simulink model "NeuromuscularModelwReflex2"  (R2019b)
settings: Solver=ode15s  StartTime=0.0  StopTime=20  MaxStep=.01  RelTol=1e-4  AbsTol=1e-6  EnableMultiTasking=on
undefined symbols (not defined in the file): footCenterToCGDist, footInertia, footMass, g, LceOffsetTA, legAngleTgt, LlegLengthClr, LongDelay, loptGAS, loptHAM, loptHAMCut, loptTA, lslackGAS, lslackHAM, lslackHAMCut, MidDelay, phimaxGASa, phimaxGASk, phimaxHAMk, phirefGASa, phirefGASk, phirefHAMh, phirefHAMk, rGASa, rGASk, rHAMh, rHAMk, rhoGASa, rhoGASk, rhoHAMh, rhoHAMk, RlegLengthClr, ShortDelay, simbiconGainD, simbiconGainV, simbiconLegAngle0, X, Y, Z
libraries: NeuroMuscularLibrary x81, nesl_utility x16, sm_lib x14, simulink x5, simulink_extras x2
(part 2 of 2)

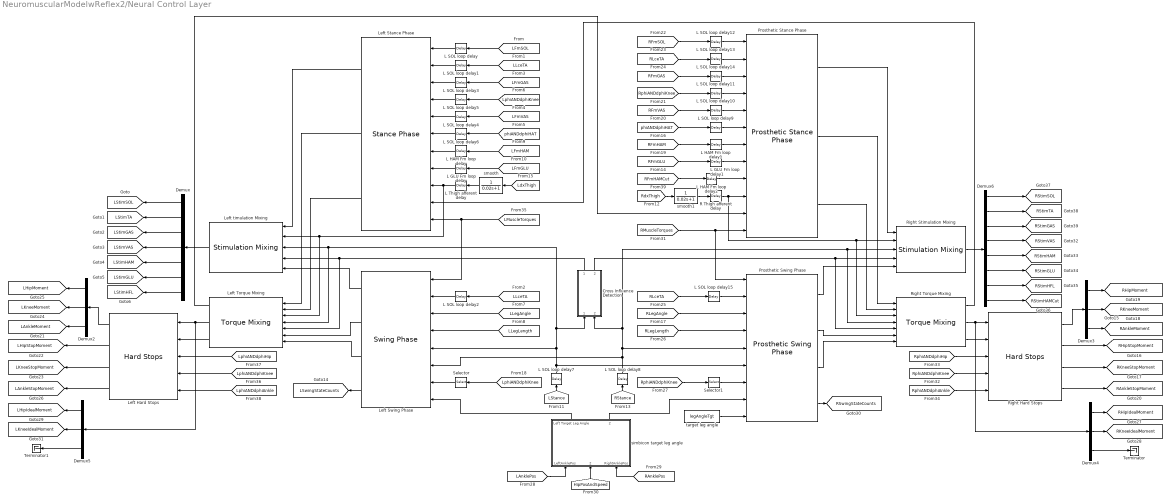
== system NeuromuscularModelwReflex2/Neural Control Layer ==
  Cross Influence Detection : Subsystem
  Demux : Demux  Outputs=7
  Demux{2..5} (4 alike) : Demux  Outputs=3
  Demux6 : Demux  Outputs=8
  L GLU Fm loop delay : TransportDelay  DelayTime=ShortDelay
  L GLU Fm loop delay1 : TransportDelay  DelayTime=ShortDelay
  L HAM Fm loop delay : TransportDelay  DelayTime=ShortDelay
  L HAM Fm loop delay1 : TransportDelay  DelayTime=ShortDelay
  L HAM Fm loop delay2 : TransportDelay  DelayTime=ShortDelay  BufferSize=2048
  L SOL loop delay{,1..3,12..15} (8 alike) : TransportDelay  DelayTime=LongDelay
  L SOL loop delay{4..5,7..8,10..11} (6 alike) : TransportDelay  DelayTime=MidDelay
  L SOL loop delay6 : TransportDelay  DelayTime=ShortDelay
  L SOL loop delay9 : TransportDelay  DelayTime=ShortDelay
  L Thigh afferent delay : TransportDelay  DelayTime=ShortDelay
  Left Hard Stops : NeuroMuscularLibrary/Hard Stops  SystemSampleTime=-1  Latency=0  AutoFrameSizeCalculation=off
  Left Stance Phase : NeuroMuscularLibrary/Stance Phase  GainHAM=LGainHAM  GainGLU=LGainGLU  GainSOL=LGainSOL  GainSOLTA=LGainSOLTA  GainTA=LGainTA  GainGAS=LGainGAS  GainVAS=LGainVAS  GainKneeOverExt=LGainKneeOverExt  PosGainGG=LPosGainGG  SpeedGainGG=LSpeedGainGG  Kglu=LKglu
  Left Swing Phase : NeuroMuscularLibrary/Swing Phase  GainTA=LGainTA  hipPGain=LhipPGain  hipDGain=LhipDGain  legAngleFilter=LlegAngleFilter  kneeFlexGain=LkneeFlexGain  kneeHoldGain1=LkneeHoldGain1  kneeHoldGain2=LkneeHoldGain2  kneeStopGain=LkneeStopGain  kneeExtendGain=LkneeExtendGain  legLengthClr=LlegLengthClr
  Left Torque Mixing : NeuroMuscularLibrary/Torque Mixing  SystemSampleTime=-1  Latency=0  AutoFrameSizeCalculation=off
  Left timulation Mixing : NeuroMuscularLibrary/Stimulation Mixing  SystemSampleTime=-1  Latency=0  AutoFrameSizeCalculation=off
  Prosthetic Stance Phase : NeuroMuscularLibrary/Prosthetic Stance Phase  GainHAM=RGainHAM  GainHAMCut=RGainHAMCut  GainGLU=RGainGLU  GainSOL=RGainSOL  GainSOLTA=RGainSOLTA  GainTA=RGainTA  GainGAS=RGainGAS  GainVAS=RGainVAS  GainKneeOverExt=RGainKneeOverExt  PosGainGG=RPosGainGG  SpeedGainGG=RSpeedGainGG  Kglu=RKglu
  Prosthetic Swing Phase : NeuroMuscularLibrary/Prosthetic Swing Phase  GainTA=RGainTA  hipPGain=RhipPGain  hipDGain=RhipDGain  legAngleFilter=RlegAngleFilter  kneeFlexGain=RkneeFlexGain  kneeHoldGain1=RkneeHoldGain1  kneeHoldGain2=RkneeHoldGain2  kneeStopGain=RkneeStopGain  kneeExtendGain=RkneeExtendGain  legLengthClr=RlegLengthClr
  R Thigh afferent delay : TransportDelay  DelayTime=ShortDelay
  Right Hard Stops : NeuroMuscularLibrary/Hard Stops  SystemSampleTime=-1  Latency=0  AutoFrameSizeCalculation=off
  Right Stimulation Mixing : NeuroMuscularLibrary/Stimulation Mixing  SystemSampleTime=-1  Latency=0  AutoFrameSizeCalculation=off
  Right Torque Mixing : NeuroMuscularLibrary/Torque Mixing  SystemSampleTime=-1  Latency=0  AutoFrameSizeCalculation=off
  Selector : Selector  InputPortWidth=2  IndexOptions=Index vector (dialog)  Indices=2  OutputSizes=1
  Selector1 : Selector  InputPortWidth=2  IndexOptions=Index vector (dialog)  Indices=2  OutputSizes=1
  Terminator : Terminator
  Terminator1 : Terminator
  simbicon target leg angle : Subsystem
  smooth : TransferFcn  Denominator=[0.02 1]
  smooth1 : TransferFcn  Denominator=[0.02 1]
  target leg angle : Constant  Value=legAngleTgt
  tag scope: LAnkleMoment=global, LAnkleStopMoment=global, LHipIdealMoment=global, LHipMoment=global, LHipStopMoment=global, LKneeIdealMoment=global, LKneeMoment=global, LKneeStopMoment=global, LStimGAS=global, LStimGLU=global, LStimHAM=global, LStimHFL=global, LStimSOL=global, LStimTA=global, LStimVAS=global, LSwingStateCounts=global, RAnkleMoment=global, RAnkleStopMoment=global, RHipIdealMoment=global, RHipMoment=global, RHipStopMoment=global, RKneeIdealMoment=global, RKneeMoment=global, RKneeStopMoment=global, RStimGAS=global, RStimGLU=global, RStimHAM=global, RStimHAMCut=global, RStimHFL=global, RStimSOL=global, RStimTA=global, RStimVAS=global, RSwingStateCounts=global
  wires:
  [LFmSOL] -> L SOL loop delay/1
  L SOL loop delay/1 -> Left Stance Phase/1
  [LLceTA] -> L SOL loop delay1/1
  L SOL loop delay1/1 -> Left Stance Phase/2
  Demux/1 -> [LStimSOL]
  Demux/2 -> [LStimTA]
  Demux/3 -> [LStimGAS]
  [LFmGAS] -> L SOL loop delay3/1
  L SOL loop delay3/1 -> Left Stance Phase/3
  [LLceTA] -> L SOL loop delay2/1
  L SOL loop delay4/1 -> Left Stance Phase/5
  [LFmVAS] -> L SOL loop delay4/1
  L SOL loop delay5/1 -> Left Stance Phase/4
  [LphiANDdphiKnee] -> L SOL loop delay5/1
  Demux/4 -> [LStimVAS]
  [phiANDdphiHAT] -> L SOL loop delay6/1
  L SOL loop delay6/1 -> Left Stance Phase/6
  Demux/5 -> [LStimHAM]
  Demux/6 -> [LStimGLU]
  Demux/7 -> [LStimHFL]
  [LdxThigh] -> smooth/1
  smooth/1 -> L Thigh afferent delay/1
  [RdxThigh] -> smooth1/1
  smooth1/1 -> R Thigh afferent delay/1
  [LFmHAM] -> L HAM Fm loop delay/1
  [LFmGLU] -> L GLU Fm loop delay/1
  L SOL loop delay7/1 -> Prosthetic Swing Phase/6, Left Swing Phase/5, Left Torque Mixing/4, Left timulation Mixing/3, Cross Influence Detection/1(LStance)
  [RFmHAM] -> L HAM Fm loop delay1/1
  [RFmGLU] -> L GLU Fm loop delay1/1
  [phiANDdphiHAT] -> L SOL loop delay9/1
  L SOL loop delay9/1 -> Prosthetic Stance Phase/6
  [LStance] -> L SOL loop delay7/1
  [RStance] -> L SOL loop delay8/1
  [RFmVAS] -> L SOL loop delay10/1
  [RphiANDdphiKnee] -> L SOL loop delay11/1
  L SOL loop delay10/1 -> Prosthetic Stance Phase/5
  L SOL loop delay11/1 -> Prosthetic Stance Phase/4
  L SOL loop delay12/1 -> Prosthetic Stance Phase/1
  [RFmSOL] -> L SOL loop delay12/1
  [RLceTA] -> L SOL loop delay13/1
  L SOL loop delay13/1 -> Prosthetic Stance Phase/2
  [RFmGAS] -> L SOL loop delay14/1
  L SOL loop delay14/1 -> Prosthetic Stance Phase/3
  [RLceTA] -> L SOL loop delay15/1
  L Thigh afferent delay/1 -> Left Torque Mixing/3, Left timulation Mixing/2, Left Stance Phase/9
  L HAM Fm loop delay/1 -> Left Stance Phase/7
  L GLU Fm loop delay/1 -> Left Stance Phase/8
  R Thigh afferent delay/1 -> Prosthetic Stance Phase/10, Right Torque Mixing/3, Right Stimulation Mixing/2
  L SOL loop delay15/1 -> Prosthetic Swing Phase/2
  L SOL loop delay2/1 -> Left Swing Phase/2
  Prosthetic Stance Phase/1 -> Right Stimulation Mixing/1
  L SOL loop delay8/1 -> Left Swing Phase/6, Prosthetic Swing Phase/5, Right Torque Mixing/4, Right Stimulation Mixing/3, Cross Influence Detection/2(RStance)
  Cross Influence Detection/2(LeftLeading) -> Right Torque Mixing/5, Right Stimulation Mixing/4
  Left timulation Mixing/1 -> Demux/1
  Left Stance Phase/1 -> Left timulation Mixing/1
  Cross Influence Detection/1(RightLeading) -> Left Torque Mixing/5, Left timulation Mixing/4
  Demux3/1 -> [RHipMoment]
  Demux3/2 -> [RKneeMoment]
  [LLegAngle] -> Left Swing Phase/3
  [LLegLength] -> Left Swing Phase/4
  [RLegAngle] -> Prosthetic Swing Phase/3
  [RLegLength] -> Prosthetic Swing Phase/4
  [RphiANDdphiKnee] -> Selector1/1
  Selector1/1 -> Prosthetic Swing Phase/7
  [LAnklePos] -> simbicon target leg angle/1(LeftAnklePos)
  [RAnklePos] -> simbicon target leg angle/3(RightAnklePos)
  Prosthetic Swing Phase/1 -> Right Stimulation Mixing/5
  [LphiANDdphiKnee] -> Selector/1
  Selector/1 -> Left Swing Phase/7
  Left Swing Phase/1 -> Left timulation Mixing/5
  [HipPosAndSpeed] -> simbicon target leg angle/2(HIPposAndSpeed)
  simbicon target leg angle/2(Right Target Leg Angle) -> Prosthetic Swing Phase/8
  simbicon target leg angle/1(Left Target Leg Angle) -> Left Swing Phase/8
  Prosthetic Swing Phase/4 -> [RSwingStateCounts]
  Left Swing Phase/4 -> [LSwingStateCounts]
  Demux3/3 -> [RAnkleMoment]
  [RphiANDdphiKnee] -> Right Hard Stops/4
  [RphiANDdphiHip] -> Right Hard Stops/3
  [RphiANDdphiAnkle] -> Right Hard Stops/5
  Right Hard Stops/2 -> [RHipStopMoment]
  Right Hard Stops/3 -> [RKneeStopMoment]
  Right Hard Stops/4 -> [RAnkleStopMoment]
  [LMuscleTorques] -> Left Swing Phase/1, Left Stance Phase/11
  Demux2/1 -> [LHipMoment]
  Demux2/3 -> [LAnkleMoment]
  Left Hard Stops/1 -> Demux2/1
  [LphiANDdphiKnee] -> Left Hard Stops/4
  [LphiANDdphiHip] -> Left Hard Stops/3
  Left Hard Stops/2 -> [LHipStopMoment]
  Left Hard Stops/3 -> [LKneeStopMoment]
  Left Hard Stops/4 -> [LAnkleStopMoment]
  Left Stance Phase/2 -> Left Torque Mixing/1
  Demux2/2 -> [LKneeMoment]
  Right Torque Mixing/2 -> Demux4/1, Right Hard Stops/1
  Right Hard Stops/1 -> Demux3/1
  [RMuscleTorques] -> Prosthetic Stance Phase/12, Prosthetic Swing Phase/1
  Demux4/1 -> [RHipIdealMoment]
  Demux4/2 -> [RKneeIdealMoment]
  Demux4/3 -> Terminator/1
  Prosthetic Swing Phase/3 -> Right Torque Mixing/7
  Prosthetic Swing Phase/2 -> Right Torque Mixing/6
  Prosthetic Stance Phase/3 -> Right Torque Mixing/2
  Prosthetic Stance Phase/2 -> Right Torque Mixing/1
  Right Torque Mixing/3 -> Right Hard Stops/2
  Right Torque Mixing/1 -> Left Stance Phase/10
  [LphiANDdphiAnkle] -> Left Hard Stops/5
  Left Torque Mixing/2 -> Demux5/1, Left Hard Stops/1
  Left Torque Mixing/3 -> Left Hard Stops/2
  Left Torque Mixing/1 -> Prosthetic Stance Phase/11
  Left Stance Phase/3 -> Left Torque Mixing/2
  Left Swing Phase/2 -> Left Torque Mixing/6
  Left Swing Phase/3 -> Left Torque Mixing/7
  Demux5/1 -> [LHipIdealMoment]
  Demux5/2 -> [LKneeIdealMoment]
  Demux5/3 -> Terminator1/1
  Demux6/1 -> [RStimSOL]
  Demux6/2 -> [RStimTA]
  Demux6/4 -> [RStimVAS]
  Demux6/5 -> [RStimHAM]
  Demux6/7 -> [RStimHFL]
  Demux6/3 -> [RStimGAS]
  Demux6/6 -> [RStimGLU]
  Right Stimulation Mixing/1 -> Demux6/1
  Demux6/8 -> [RStimHAMCut]
  L HAM Fm loop delay1/1 -> Prosthetic Stance Phase/7
  L GLU Fm loop delay1/1 -> Prosthetic Stance Phase/8
  [RFmHAMCut] -> L HAM Fm loop delay2/1
  L HAM Fm loop delay2/1 -> Prosthetic Stance Phase/9
  target leg angle/1 -> Prosthetic Swing Phase/9

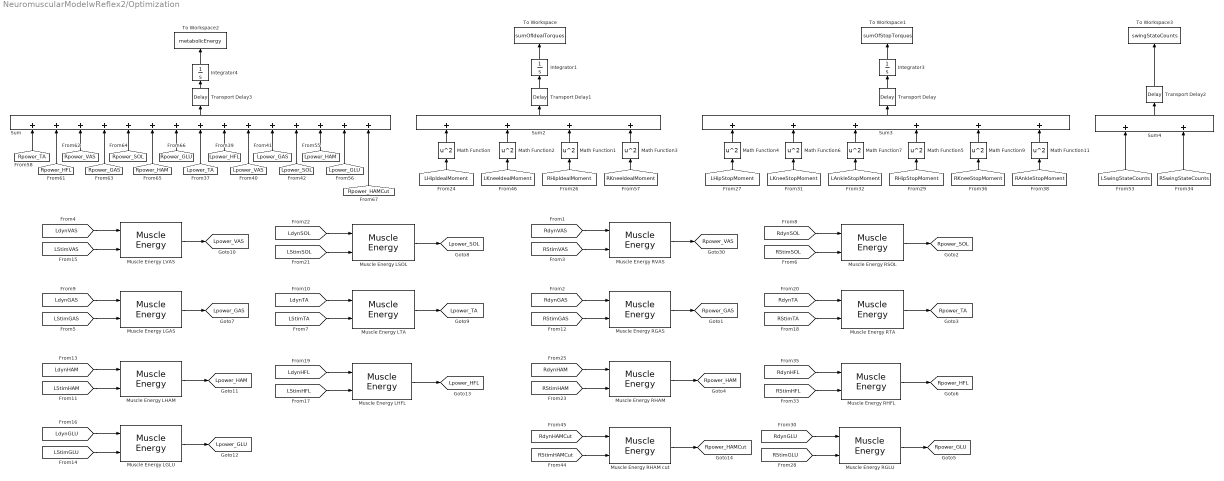
== system NeuromuscularModelwReflex2/Optimization ==
  Integrator1 : Integrator
  Integrator3 : Integrator
  Integrator4 : Integrator
  Math Function{,1..7,9,11} (10 alike) : Math  Operator=square  SaturateOnIntegerOverflow=on
  Muscle Energy LGAS : NeuroMuscularLibrary/Muscle Energy  lopt=loptGAS  FT=FT_GAS  Fmax=FmaxGAS
  Muscle Energy LGLU : NeuroMuscularLibrary/Muscle Energy  lopt=loptGLU  FT=FT_GLU  Fmax=FmaxGLU
  Muscle Energy LHAM : NeuroMuscularLibrary/Muscle Energy  lopt=loptHAM  FT=FT_HAM  Fmax=FmaxHAM
  Muscle Energy LHFL : NeuroMuscularLibrary/Muscle Energy  lopt=loptHFL  FT=FT_HFL  Fmax=FmaxHFL
  Muscle Energy LSOL : NeuroMuscularLibrary/Muscle Energy  lopt=loptSOL  FT=FT_SOL  Fmax=FmaxSOL
  Muscle Energy LTA : NeuroMuscularLibrary/Muscle Energy  lopt=loptTA  FT=FT_TA  Fmax=FmaxTA
  Muscle Energy LVAS : NeuroMuscularLibrary/Muscle Energy  lopt=loptVAS  FT=FT_VAS  Fmax=FmaxVAS
  Muscle Energy RGAS : NeuroMuscularLibrary/Muscle Energy  lopt=loptGAS  FT=FT_GAS  Fmax=FmaxGAS
  Muscle Energy RGLU : NeuroMuscularLibrary/Muscle Energy  lopt=loptGLU  FT=FT_GLU  Fmax=FmaxGLU
  Muscle Energy RHAM : NeuroMuscularLibrary/Muscle Energy  lopt=loptHAM  FT=FT_HAM  Fmax=FmaxHAM
  Muscle Energy RHAM cut : NeuroMuscularLibrary/Muscle Energy  lopt=loptHAMCut  FT=FT_HAM  Fmax=FmaxHAMCut
  Muscle Energy RHFL : NeuroMuscularLibrary/Muscle Energy  lopt=loptHFL  FT=FT_HFL  Fmax=FmaxHFL
  Muscle Energy RSOL : NeuroMuscularLibrary/Muscle Energy  lopt=loptSOL  FT=FT_SOL  Fmax=FmaxSOL
  Muscle Energy RTA : NeuroMuscularLibrary/Muscle Energy  lopt=loptTA  FT=FT_TA  Fmax=FmaxTA
  Muscle Energy RVAS : NeuroMuscularLibrary/Muscle Energy  lopt=loptVAS  FT=FT_VAS  Fmax=FmaxVAS
  Sum : Sum  Inputs=+++++++++++++++
  Sum2 : Sum  Inputs=++++
  Sum3 : Sum  Inputs=++++++
  Sum4 : Sum
  To Workspace : ToWorkspace  VariableName=sumOfIdealTorques  SampleTime=-1
      settings: MaxDataPoints=1
  To Workspace1 : ToWorkspace  VariableName=sumOfStopTorques  SampleTime=-1
      settings: MaxDataPoints=1
  To Workspace2 : ToWorkspace  VariableName=metabolicEnergy  SampleTime=-1
      settings: MaxDataPoints=1
  To Workspace3 : ToWorkspace  VariableName=swingStateCounts  SampleTime=-1
      settings: MaxDataPoints=1
  Transport Delay{,1..3} (4 alike) : TransportDelay  DelayTime=3  BufferSize=24576
  tag scope: Lpower_GAS=global, Lpower_GLU=global, Lpower_HAM=global, Lpower_HFL=global, Lpower_SOL=global, Lpower_TA=global, Lpower_VAS=global, Rpower_GAS=global, Rpower_GLU=global, Rpower_HAM=global, Rpower_HAMCut=global, Rpower_HFL=global, Rpower_SOL=global, Rpower_TA=global, Rpower_VAS=global
  wires:
  [RdynSOL] -> Muscle Energy RSOL/1
  [RStimSOL] -> Muscle Energy RSOL/2
  [RStimVAS] -> Muscle Energy RVAS/2
  [RStimGAS] -> Muscle Energy RGAS/2
  Muscle Energy RVAS/1 -> [Rpower_VAS]
  Muscle Energy RGAS/1 -> [Rpower_GAS]
  Muscle Energy RSOL/1 -> [Rpower_SOL]
  Muscle Energy RTA/1 -> [Rpower_TA]
  [RdynTA] -> Muscle Energy RTA/1
  [RStimTA] -> Muscle Energy RTA/2
  [RdynHAM] -> Muscle Energy RHAM/1
  [RStimHAM] -> Muscle Energy RHAM/2
  [RdynGLU] -> Muscle Energy RGLU/1
  [RStimGLU] -> Muscle Energy RGLU/2
  [RdynHFL] -> Muscle Energy RHFL/1
  [RStimHFL] -> Muscle Energy RHFL/2
  Muscle Energy RHAM/1 -> [Rpower_HAM]
  Muscle Energy RGLU/1 -> [Rpower_GLU]
  Muscle Energy RHFL/1 -> [Rpower_HFL]
  [RdynGAS] -> Muscle Energy RGAS/1
  [RdynVAS] -> Muscle Energy RVAS/1
  [LdynSOL] -> Muscle Energy LSOL/1
  [LStimSOL] -> Muscle Energy LSOL/2
  [LStimVAS] -> Muscle Energy LVAS/2
  [LStimGAS] -> Muscle Energy LGAS/2
  Muscle Energy LVAS/1 -> [Lpower_VAS]
  Muscle Energy LGAS/1 -> [Lpower_GAS]
  Muscle Energy LSOL/1 -> [Lpower_SOL]
  Muscle Energy LTA/1 -> [Lpower_TA]
  [LdynTA] -> Muscle Energy LTA/1
  [LStimTA] -> Muscle Energy LTA/2
  [LdynHAM] -> Muscle Energy LHAM/1
  [LStimHAM] -> Muscle Energy LHAM/2
  [LdynGLU] -> Muscle Energy LGLU/1
  [LStimGLU] -> Muscle Energy LGLU/2
  [LdynHFL] -> Muscle Energy LHFL/1
  [LStimHFL] -> Muscle Energy LHFL/2
  Muscle Energy LHAM/1 -> [Lpower_HAM]
  Muscle Energy LGLU/1 -> [Lpower_GLU]
  Muscle Energy LHFL/1 -> [Lpower_HFL]
  [LdynGAS] -> Muscle Energy LGAS/1
  [LdynVAS] -> Muscle Energy LVAS/1
  [RdynHAMCut] -> Muscle Energy RHAM cut/1
  [RStimHAMCut] -> Muscle Energy RHAM cut/2
  Muscle Energy RHAM cut/1 -> [Rpower_HAMCut]
  Integrator1/1 -> To Workspace/1
  Math Function/1 -> Sum2/1
  [LHipIdealMoment] -> Math Function/1
  Math Function2/1 -> Sum2/2
  [LKneeIdealMoment] -> Math Function2/1
  [RHipIdealMoment] -> Math Function1/1
  Math Function1/1 -> Sum2/3
  [RKneeIdealMoment] -> Math Function3/1
  Math Function3/1 -> Sum2/4
  Integrator3/1 -> To Workspace1/1
  Math Function4/1 -> Sum3/1
  [LHipStopMoment] -> Math Function4/1
  Math Function6/1 -> Sum3/2
  [LKneeStopMoment] -> Math Function6/1
  [RHipStopMoment] -> Math Function5/1
  Math Function7/1 -> Sum3/3
  [LAnkleStopMoment] -> Math Function7/1
  Sum3/1 -> Transport Delay/1
  Transport Delay/1 -> Integrator3/1
  [RKneeStopMoment] -> Math Function9/1
  Math Function9/1 -> Sum3/5
  [RAnkleStopMoment] -> Math Function11/1
  Math Function11/1 -> Sum3/6
  Sum4/1 -> Transport Delay2/1
  Transport Delay2/1 -> To Workspace3/1
  [LSwingStateCounts] -> Sum4/1
  [RSwingStateCounts] -> Sum4/2
  [Rpower_TA] -> Sum/1
  [Rpower_GLU] -> Sum/7
  [Rpower_HAM] -> Sum/6
  [Rpower_SOL] -> Sum/5
  [Rpower_GAS] -> Sum/4
  [Rpower_VAS] -> Sum/3
  [Rpower_HFL] -> Sum/2
  [Lpower_TA] -> Sum/8
  [Lpower_GLU] -> Sum/14
  [Lpower_HAM] -> Sum/13
  [Lpower_SOL] -> Sum/12
  [Lpower_GAS] -> Sum/11
  [Lpower_VAS] -> Sum/10
  [Lpower_HFL] -> Sum/9
  Integrator4/1 -> To Workspace2/1
  Sum/1 -> Transport Delay3/1
  Transport Delay3/1 -> Integrator4/1
  [Rpower_HAMCut] -> Sum/15
  Sum2/1 -> Transport Delay1/1
  Transport Delay1/1 -> Integrator1/1
  Math Function5/1 -> Sum3/4

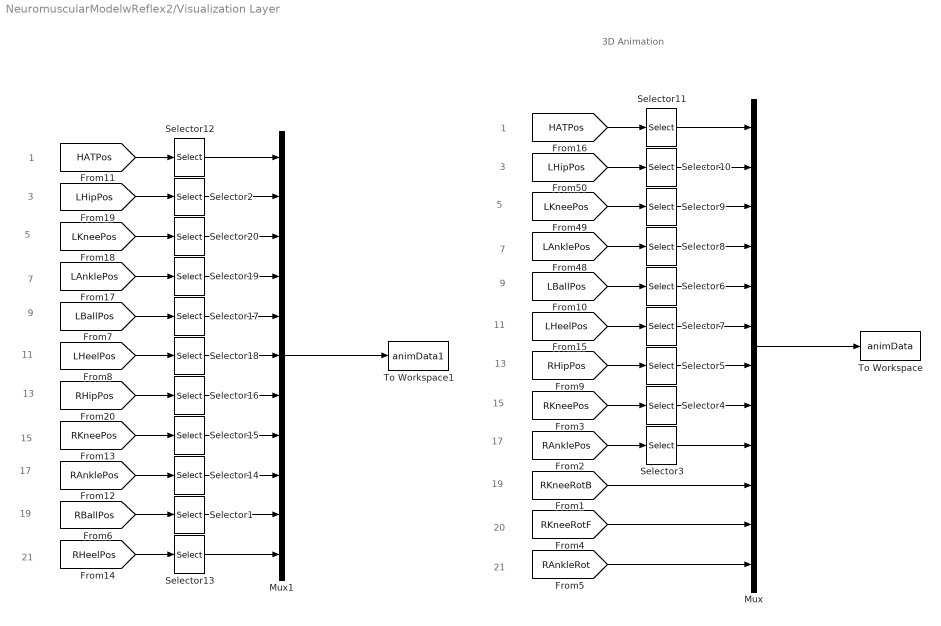
== system NeuromuscularModelwReflex2/Visualization Layer ==
  note: 20
  note: 19
  note: 17
  note: 15
  note: 13
  note: 11
  note: 9
  note: 7
  note: 5
  note: 3
  note: 1
  note: 3D Animation
  note: 21
  note: 5
  note: 17
  note: 19
  note: 15
  note: 9
  note: 1
  note: 7
  note: 21
  note: 11
  note: 3
  note: 13
  Mux : Mux  Inputs=12
  Mux1 : Mux  Inputs=11
  Selector{1..20} (20 alike) : Selector  InputPortWidth=3  IndexOptions=Index vector (dialog)  Indices=[1 3]  OutputSizes=1
  To Workspace : ToWorkspace  VariableName=animData  SaveFormat=Structure With Time  SampleTime=1/30
  To Workspace1 : ToWorkspace  VariableName=animData1  SaveFormat=Structure With Time  SampleTime=1/30
  wires:
  [RAnklePos] -> Selector3/1
  [RKneePos] -> Selector4/1
  [RHipPos] -> Selector5/1
  [HATPos] -> Selector11/1
  [LHeelPos] -> Selector7/1
  [LBallPos] -> Selector6/1
  [LAnklePos] -> Selector8/1
  [LKneePos] -> Selector9/1
  [LHipPos] -> Selector10/1
  Selector11/1 -> Mux/1
  Selector3/1 -> Mux/9
  Selector4/1 -> Mux/8
  Selector5/1 -> Mux/7
  Selector7/1 -> Mux/6
  Selector6/1 -> Mux/5
  Selector8/1 -> Mux/4
  Selector9/1 -> Mux/3
  Selector10/1 -> Mux/2
  [RKneeRotB] -> Mux/10
  [RKneeRotF] -> Mux/11
  [RAnkleRot] -> Mux/12
  Mux/1 -> To Workspace/1
  Mux1/1 -> To Workspace1/1
  Selector13/1 -> Mux1/11
  Selector15/1 -> Mux1/8
  Selector1/1 -> Mux1/10
  [RAnklePos] -> Selector14/1
  Selector20/1 -> Mux1/3
  [RBallPos] -> Selector1/1
  Selector18/1 -> Mux1/6
  [LKneePos] -> Selector20/1
  [HATPos] -> Selector12/1
  Selector12/1 -> Mux1/1
  [RKneePos] -> Selector15/1
  [LBallPos] -> Selector17/1
  [LHeelPos] -> Selector18/1
  Selector17/1 -> Mux1/5
  [LAnklePos] -> Selector19/1
  Selector2/1 -> Mux1/2
  [RHeelPos] -> Selector13/1
  [LHipPos] -> Selector2/1
  Selector19/1 -> Mux1/4
  Selector14/1 -> Mux1/9
  [RHipPos] -> Selector16/1
  Selector16/1 -> Mux1/7

== system NeuromuscularModelwReflex2/Body Mechanics Layer/HAT Speed Sensor ==
  PS-Simulink Converter1 : nesl_utility/PS-Simulink Converter  PhysicalDomain=network_engine_domain  SubClassName=ps_output  LeftPortType=input  RightPortType=output  PseudoPeriodic=off  Frequencies=[]  Unit=m/s  AffineConversion=off
  Position Sensor : sm_lib/Frames and Transforms/Transform Sensor  MeasurementFrame=World  SenseAngle=off  SenseAxis=off  SenseAngle1=off  SenseAngle2=off  SenseAngle3=off  SenseQ=off  SenseR=off  SenseOmegaX=off  SenseOmegaY=off  SenseOmegaZ=off  SenseOmega1=off  SenseOmega2=off  SenseOmega3=off  SenseQDot=off  SenseRDot=off  SenseAlphaX=off  SenseAlphaY=off  SenseAlphaZ=off  SenseAlpha1=off  SenseAlpha2=off  SenseAlpha3=off  SenseQDDot=off  SenseRDDot=off  SenseX=off  SenseY=off  SenseZ=off  SenseRad=off  SenseAzim=off  SenseDist=off  SenseInc=off  SenseXDot=on  SenseYDot=off  SenseZDot=off  SenseRadDot=off  SenseAzimDot=off  SenseDistDot=off  SenseIncDot=off  SenseXDDot=off  SenseYDDot=off  SenseZDDot=off  SenseRadDDot=off  SenseAzimDDot=off  SenseDistDDot=off  SenseIncDDot=off
  World Frame : sm_lib/Frames and Transforms/World Frame
  Frame : PMIOPort  Side=Left
  Speed : Outport
  wires:
  PS-Simulink Converter1/1 -> Speed/1
  connections:
  Position Sensor/LConn1 -- World Frame/RConn1
  Position Sensor/RConn1 -- Frame/RConn1
  Position Sensor/RConn2 -- PS-Simulink Converter1/LConn1

== system NeuromuscularModelwReflex2/Body Mechanics Layer/Hip Pos//Speed Sensor ==
  Mux : Mux  Inputs=2
  PS-Simulink Converter : nesl_utility/PS-Simulink Converter  PhysicalDomain=network_engine_domain  SubClassName=ps_output  LeftPortType=input  RightPortType=output  PseudoPeriodic=off  Frequencies=[]  Unit=m  AffineConversion=off
  PS-Simulink Converter1 : nesl_utility/PS-Simulink Converter  PhysicalDomain=network_engine_domain  SubClassName=ps_output  LeftPortType=input  RightPortType=output  PseudoPeriodic=off  Frequencies=[]  Unit=m/s  AffineConversion=off
  Position Sensor : sm_lib/Frames and Transforms/Transform Sensor  MeasurementFrame=World  SenseAngle=off  SenseAxis=off  SenseAngle1=off  SenseAngle2=off  SenseAngle3=off  SenseQ=off  SenseR=off  SenseOmegaX=off  SenseOmegaY=off  SenseOmegaZ=off  SenseOmega1=off  SenseOmega2=off  SenseOmega3=off  SenseQDot=off  SenseRDot=off  SenseAlphaX=off  SenseAlphaY=off  SenseAlphaZ=off  SenseAlpha1=off  SenseAlpha2=off  SenseAlpha3=off  SenseQDDot=off  SenseRDDot=off  SenseX=on  SenseY=off  SenseZ=off  SenseRad=off  SenseAzim=off  SenseDist=off  SenseInc=off  SenseXDot=on  SenseYDot=off  SenseZDot=off  SenseRadDot=off  SenseAzimDot=off  SenseDistDot=off  SenseIncDot=off  SenseXDDot=off  SenseYDDot=off  SenseZDDot=off  SenseRadDDot=off  SenseAzimDDot=off  SenseDistDDot=off  SenseIncDDot=off
  World Frame : sm_lib/Frames and Transforms/World Frame
  Frame : PMIOPort  Side=Left
  PosSpeed : Outport
  wires:
  Mux/1 -> PosSpeed/1
  PS-Simulink Converter/1 -> Mux/1
  PS-Simulink Converter1/1 -> Mux/2
  connections:
  Position Sensor/LConn1 -- World Frame/RConn1
  Position Sensor/RConn1 -- Frame/RConn1
  PS-Simulink Converter/LConn1 -- Position Sensor/RConn2
  PS-Simulink Converter1/LConn1 -- Position Sensor/RConn3

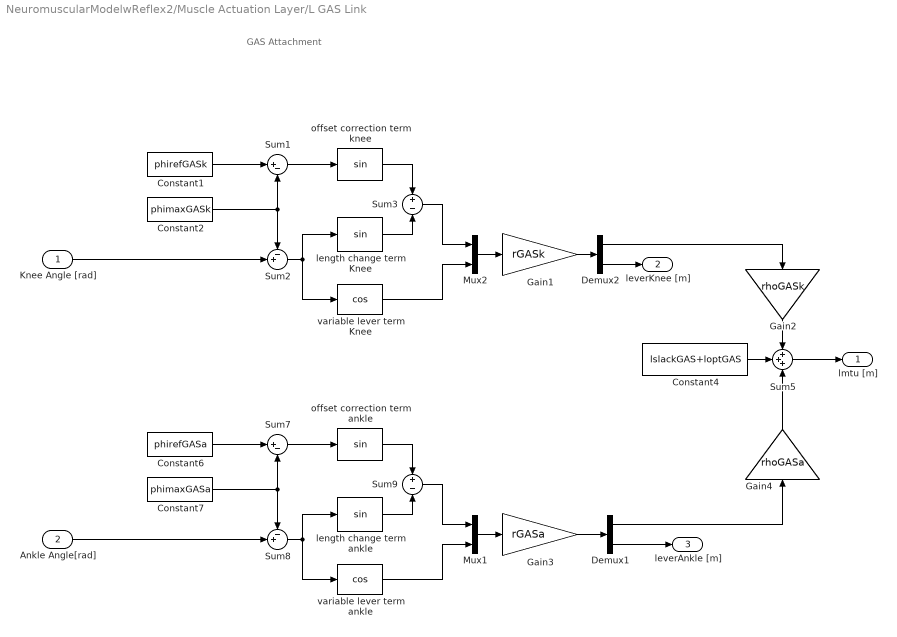
== system NeuromuscularModelwReflex2/Muscle Actuation Layer/L GAS Link ==
  note: GAS Attachment
  Knee Angle [rad] : Inport
  Ankle Angle[rad] : Inport  Port=2
  Constant1 : Constant  Value=phirefGASk
  Constant2 : Constant  Value=phimaxGASk
  Constant4 : Constant  Value=lslackGAS+loptGAS
  Constant6 : Constant  Value=phirefGASa
  Constant7 : Constant  Value=phimaxGASa
  Demux1 : Demux  Outputs=2
  Demux2 : Demux  Outputs=2
  Gain1 : Gain  Gain=rGASk
  Gain2 : Gain  Gain=rhoGASk
  Gain3 : Gain  Gain=rGASa
  Gain4 : Gain  Gain=rhoGASa
  Mux1 : Mux  Inputs=2
  Mux2 : Mux  Inputs=2
  Sum1 : Sum  Inputs=|+-
  Sum2 : Sum  Inputs=-+|
  Sum3 : Sum  Inputs=+-
  Sum5 : Sum  Inputs=+++
  Sum7 : Sum  Inputs=|+-
  Sum8 : Sum  Inputs=-+|
  Sum9 : Sum  Inputs=+-
  length change term Knee : Trigonometry
  length change term ankle : Trigonometry
  offset correction term ankle : Trigonometry
  offset correction term knee : Trigonometry
  variable lever term Knee : Trigonometry  Operator=cos
  variable lever term ankle : Trigonometry  Operator=cos
  lmtu [m] : Outport
  leverKnee [m] : Outport  Port=2
  leverAnkle [m] : Outport  Port=3
  wires:
  Ankle Angle[rad]/1 -> Sum8/2
  Sum5/1 -> lmtu [m]/1
  variable lever term ankle/1 -> Mux1/2
  Demux1/2 -> leverAnkle [m]/1
  Sum8/1 -> variable lever term ankle/1, length change term ankle/1
  Constant7/1 -> Sum8/1, Sum7/2
  Sum7/1 -> offset correction term ankle/1
  Constant6/1 -> Sum7/1
  length change term ankle/1 -> Sum9/2
  offset correction term ankle/1 -> Sum9/1
  Sum9/1 -> Mux1/1
  Constant4/1 -> Sum5/2
  Mux1/1 -> Gain3/1
  Gain3/1 -> Demux1/1
  Demux1/1 -> Gain4/1
  Gain4/1 -> Sum5/3
  Knee Angle [rad]/1 -> Sum2/2
  variable lever term Knee/1 -> Mux2/2
  Sum2/1 -> variable lever term Knee/1, length change term Knee/1
  Constant2/1 -> Sum2/1, Sum1/2
  Sum1/1 -> offset correction term knee/1
  Constant1/1 -> Sum1/1
  length change term Knee/1 -> Sum3/2
  offset correction term knee/1 -> Sum3/1
  Sum3/1 -> Mux2/1
  Mux2/1 -> Gain1/1
  Gain1/1 -> Demux2/1
  Demux2/2 -> leverKnee [m]/1
  Demux2/1 -> Gain2/1
  Gain2/1 -> Sum5/1

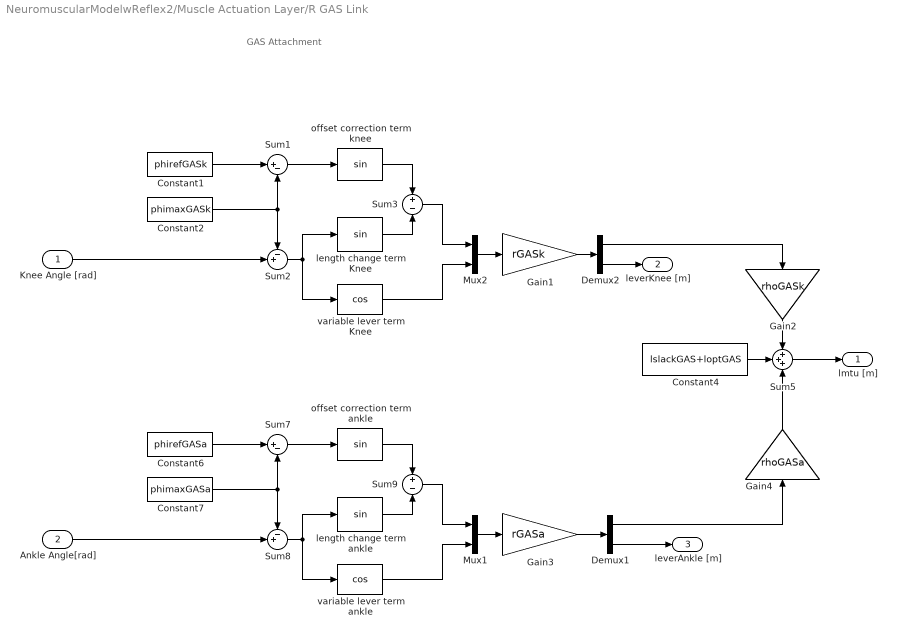
== system NeuromuscularModelwReflex2/Muscle Actuation Layer/R GAS Link ==
  note: GAS Attachment
  Knee Angle [rad] : Inport
  Ankle Angle[rad] : Inport  Port=2
  Constant1 : Constant  Value=phirefGASk
  Constant2 : Constant  Value=phimaxGASk
  Constant4 : Constant  Value=lslackGAS+loptGAS
  Constant6 : Constant  Value=phirefGASa
  Constant7 : Constant  Value=phimaxGASa
  Demux1 : Demux  Outputs=2
  Demux2 : Demux  Outputs=2
  Gain1 : Gain  Gain=rGASk
  Gain2 : Gain  Gain=rhoGASk
  Gain3 : Gain  Gain=rGASa
  Gain4 : Gain  Gain=rhoGASa
  Mux1 : Mux  Inputs=2
  Mux2 : Mux  Inputs=2
  Sum1 : Sum  Inputs=|+-
  Sum2 : Sum  Inputs=-+|
  Sum3 : Sum  Inputs=+-
  Sum5 : Sum  Inputs=+++
  Sum7 : Sum  Inputs=|+-
  Sum8 : Sum  Inputs=-+|
  Sum9 : Sum  Inputs=+-
  length change term Knee : Trigonometry
  length change term ankle : Trigonometry
  offset correction term ankle : Trigonometry
  offset correction term knee : Trigonometry
  variable lever term Knee : Trigonometry  Operator=cos
  variable lever term ankle : Trigonometry  Operator=cos
  lmtu [m] : Outport
  leverKnee [m] : Outport  Port=2
  leverAnkle [m] : Outport  Port=3
  wires:
  Ankle Angle[rad]/1 -> Sum8/2
  Sum5/1 -> lmtu [m]/1
  variable lever term ankle/1 -> Mux1/2
  Demux1/2 -> leverAnkle [m]/1
  Sum8/1 -> variable lever term ankle/1, length change term ankle/1
  Constant7/1 -> Sum8/1, Sum7/2
  Sum7/1 -> offset correction term ankle/1
  Constant6/1 -> Sum7/1
  length change term ankle/1 -> Sum9/2
  offset correction term ankle/1 -> Sum9/1
  Sum9/1 -> Mux1/1
  Constant4/1 -> Sum5/2
  Mux1/1 -> Gain3/1
  Gain3/1 -> Demux1/1
  Demux1/1 -> Gain4/1
  Gain4/1 -> Sum5/3
  Knee Angle [rad]/1 -> Sum2/2
  variable lever term Knee/1 -> Mux2/2
  Sum2/1 -> variable lever term Knee/1, length change term Knee/1
  Constant2/1 -> Sum2/1, Sum1/2
  Sum1/1 -> offset correction term knee/1
  Constant1/1 -> Sum1/1
  length change term Knee/1 -> Sum3/2
  offset correction term knee/1 -> Sum3/1
  Sum3/1 -> Mux2/1
  Mux2/1 -> Gain1/1
  Gain1/1 -> Demux2/1
  Demux2/2 -> leverKnee [m]/1
  Demux2/1 -> Gain2/1
  Gain2/1 -> Sum5/1

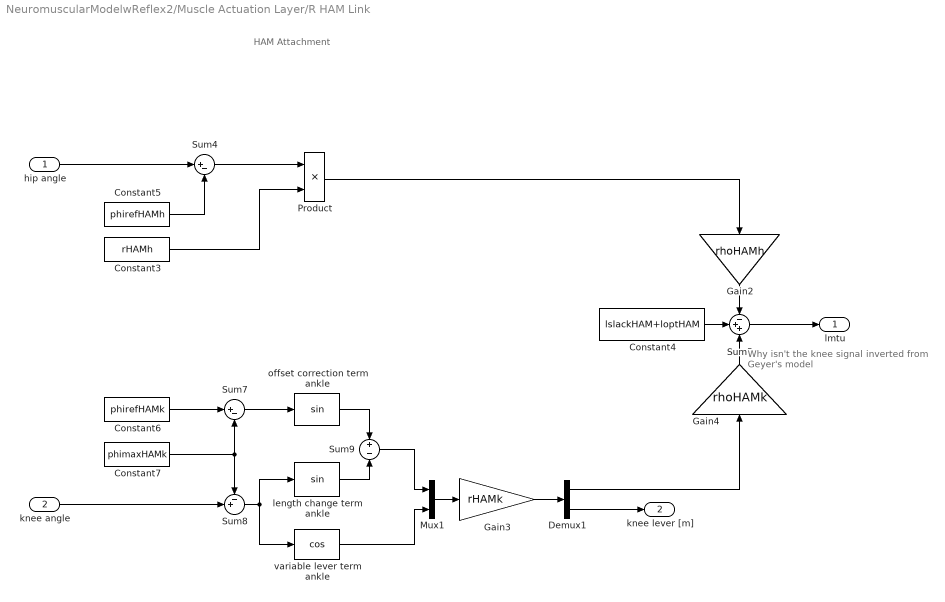
== system NeuromuscularModelwReflex2/Muscle Actuation Layer/R HAM Link ==
  note: HAM Attachment
  note: Why isn't the knee signal inverted from
      | Geyer's model
  hip angle : Inport
  knee angle : Inport  Port=2
  Constant3 : Constant  Value=rHAMh
  Constant4 : Constant  Value=lslackHAM+loptHAM
  Constant5 : Constant  Value=phirefHAMh
  Constant6 : Constant  Value=phirefHAMk
  Constant7 : Constant  Value=phimaxHAMk  VectorParams1D=off
  Demux1 : Demux  Outputs=2
  Gain2 : Gain  Gain=rhoHAMh
  Gain3 : Gain  Gain=rHAMk
  Gain4 : Gain  Gain=rhoHAMk
  Mux1 : Mux  Inputs=2
  Product : Product  RndMeth=Zero
  Sum4 : Sum  Inputs=|+-
  Sum5 : Sum  Inputs=-++
  Sum7 : Sum  Inputs=|+-
  Sum8 : Sum  Inputs=-+|
  Sum9 : Sum  Inputs=+-
  length change term ankle : Trigonometry
  offset correction term ankle : Trigonometry
  variable lever term ankle : Trigonometry  Operator=cos
  lmtu : Outport
  knee lever [m] : Outport  Port=2
  wires:
  knee angle/1 -> Sum8/2
  hip angle/1 -> Sum4/1
  Gain2/1 -> Sum5/1
  Gain4/1 -> Sum5/3
  Demux1/1 -> Gain4/1
  Gain3/1 -> Demux1/1
  Mux1/1 -> Gain3/1
  Constant4/1 -> Sum5/2
  Sum9/1 -> Mux1/1
  offset correction term ankle/1 -> Sum9/1
  length change term ankle/1 -> Sum9/2
  Constant6/1 -> Sum7/1
  Sum7/1 -> offset correction term ankle/1
  Constant7/1 -> Sum7/2, Sum8/1
  Sum8/1 -> length change term ankle/1, variable lever term ankle/1
  Demux1/2 -> knee lever [m]/1
  variable lever term ankle/1 -> Mux1/2
  Sum5/1 -> lmtu/1
  Product/1 -> Gain2/1
  Constant3/1 -> Product/2
  Sum4/1 -> Product/1
  Constant5/1 -> Sum4/2

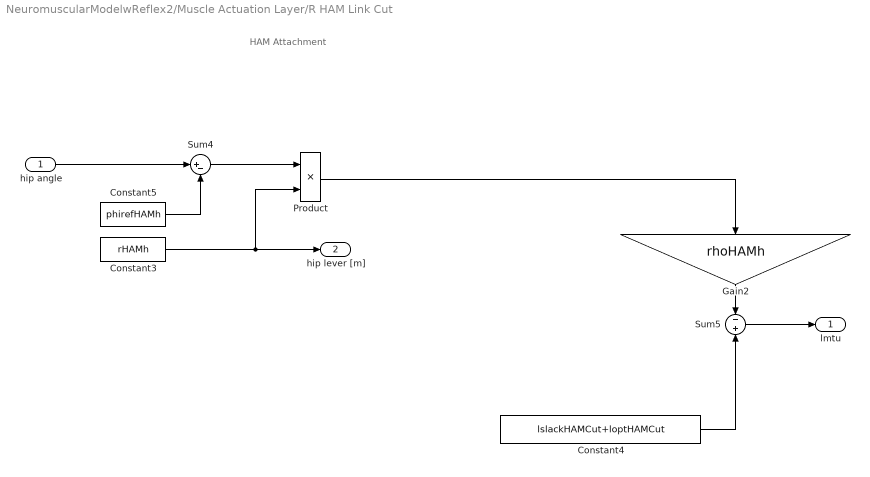
== system NeuromuscularModelwReflex2/Muscle Actuation Layer/R HAM Link Cut ==
  note: HAM Attachment
  hip angle : Inport
  Constant3 : Constant  Value=rHAMh
  Constant4 : Constant  Value=lslackHAMCut+loptHAMCut
  Constant5 : Constant  Value=phirefHAMh
  Gain2 : Gain  Gain=rhoHAMh
  Product : Product  RndMeth=Zero
  Sum4 : Sum  Inputs=|+-
  Sum5 : Sum  Inputs=-+
  lmtu : Outport
  hip lever [m] : Outport  Port=2
  wires:
  hip angle/1 -> Sum4/1
  Gain2/1 -> Sum5/1
  Constant4/1 -> Sum5/2
  Sum5/1 -> lmtu/1
  Product/1 -> Gain2/1
  Constant3/1 -> Product/2, hip lever [m]/1
  Sum4/1 -> Product/1
  Constant5/1 -> Sum4/2

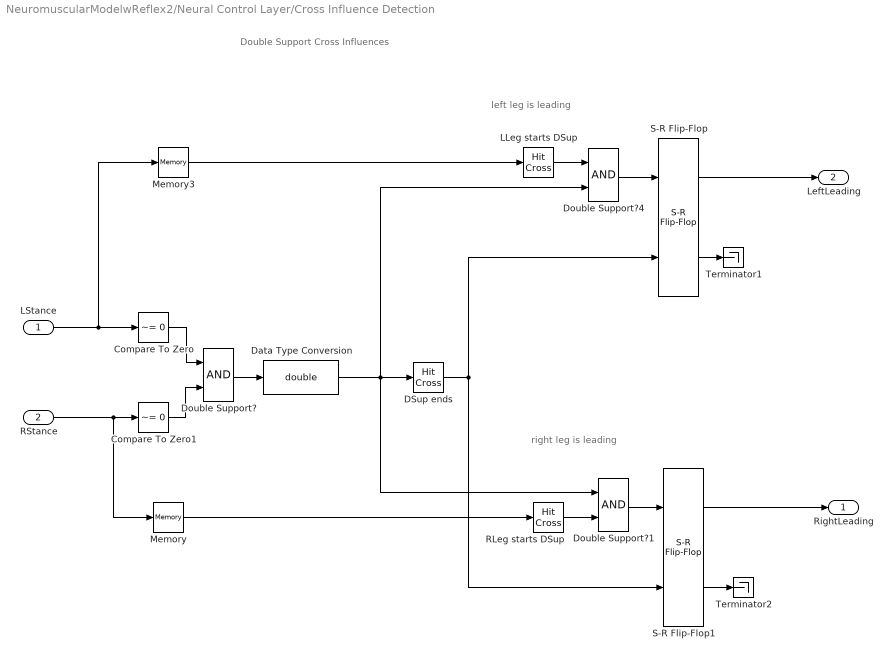
== system NeuromuscularModelwReflex2/Neural Control Layer/Cross Influence Detection ==
  note: right leg is leading
  note: left leg is leading
  note: Double Support Cross Influences
  LStance : Inport
  RStance : Inport  Port=2
  Compare To Zero : simulink/Logic and Bit Operations/Compare To Zero  relop=~=  OutDataTypeStr=boolean
  Compare To Zero1 : simulink/Logic and Bit Operations/Compare To Zero  relop=~=  OutDataTypeStr=boolean
  DSup ends : HitCross  HitCrossingOffset=0.5  HitCrossingDirection=falling  ZeroCross=off
  Data Type Conversion : DataTypeConversion  OutDataTypeStr=double
  Double Support? : Logic  AllPortsSameDT=off
  Double Support?1 : Logic  AllPortsSameDT=off
  Double Support?4 : Logic  AllPortsSameDT=off
  LLeg starts DSup : HitCross  HitCrossingOffset=0.5  HitCrossingDirection=rising  ZeroCross=off
  Memory : Memory
  Memory3 : Memory
  RLeg starts DSup : HitCross  HitCrossingOffset=0.5  HitCrossingDirection=rising  ZeroCross=off
  S-R Flip-Flop : simulink_extras/Flip Flops/S-R Flip-Flop  initial_condition=0
  S-R Flip-Flop1 : simulink_extras/Flip Flops/S-R Flip-Flop  initial_condition=0
  Terminator1 : Terminator
  Terminator2 : Terminator
  RightLeading : Outport
  LeftLeading : Outport  Port=2
  wires:
  S-R Flip-Flop/2 -> Terminator1/1
  S-R Flip-Flop/1 -> LeftLeading/1
  S-R Flip-Flop1/2 -> Terminator2/1
  LStance/1 -> Memory3/1, Compare To Zero/1
  RStance/1 -> Compare To Zero1/1, Memory/1
  S-R Flip-Flop1/1 -> RightLeading/1
  Memory/1 -> RLeg starts DSup/1
  RLeg starts DSup/1 -> Double Support?1/2
  Double Support?1/1 -> S-R Flip-Flop1/1
  Memory3/1 -> LLeg starts DSup/1
  LLeg starts DSup/1 -> Double Support?4/1
  Double Support?4/1 -> S-R Flip-Flop/1
  DSup ends/1 -> S-R Flip-Flop/2, S-R Flip-Flop1/2
  Compare To Zero/1 -> Double Support?/1
  Compare To Zero1/1 -> Double Support?/2
  Double Support?/1 -> Data Type Conversion/1
  Data Type Conversion/1 -> Double Support?1/1, Double Support?4/2, DSup ends/1

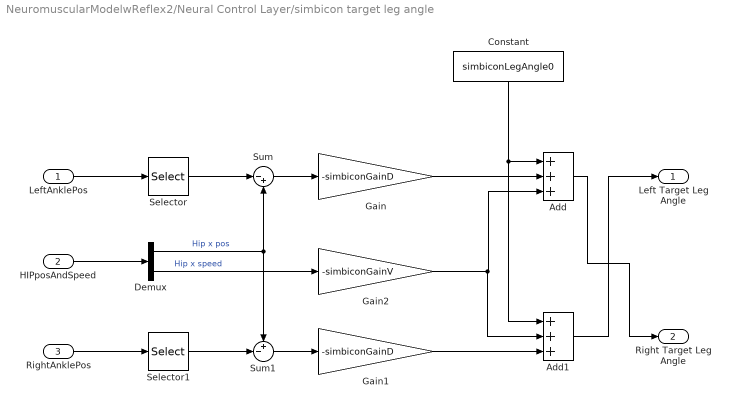
== system NeuromuscularModelwReflex2/Neural Control Layer/simbicon target leg angle ==
  LeftAnklePos : Inport
  HIPposAndSpeed : Inport  Port=2
  RightAnklePos : Inport  Port=3
  Add : Sum  Inputs=+++
  Add1 : Sum  Inputs=+++
  Constant : Constant  Value=simbiconLegAngle0
  Demux : Demux  Outputs=2
  Gain : Gain  Gain=-simbiconGainD
  Gain1 : Gain  Gain=-simbiconGainD
  Gain2 : Gain  Gain=-simbiconGainV
  Selector : Selector  InputPortWidth=3  IndexOptions=Index vector (dialog)  Indices=[1]  OutputSizes=1
  Selector1 : Selector  InputPortWidth=3  IndexOptions=Index vector (dialog)  Indices=[1]  OutputSizes=1
  Sum : Sum  Inputs=|-+
  Sum1 : Sum  Inputs=+-|
  Left Target Leg Angle : Outport
  Right Target Leg Angle : Outport  Port=2
  wires:
  HIPposAndSpeed/1 -> Demux/1
  Demux/1 -> Sum/2, Sum1/1  "Hip x pos"
  Sum/1 -> Gain/1
  Sum1/1 -> Gain1/1
  Gain/1 -> Add/2
  Gain2/1 -> Add1/2, Add/3
  Gain1/1 -> Add1/3
  Constant/1 -> Add/1, Add1/1
  Add1/1 -> Left Target Leg Angle/1
  Add/1 -> Right Target Leg Angle/1
  LeftAnklePos/1 -> Selector/1
  Selector/1 -> Sum/1
  RightAnklePos/1 -> Selector1/1
  Selector1/1 -> Sum1/2
  Demux/2 -> Gain2/1  "Hip x speed"
